simulink model "sample04_speed_pid"  (R2023a)
settings: Solver=ode1  StartTime=0.0  StopTime=inf  FixedStep=0.005  RelTol=1e-3  EnableMultiTasking=on
libraries: arduinolib x7, simulink x3, svdutilitieslib x1
settings Model: ExtModeTrigDuration=2  Creator=kawata  LastModifiedBy=kawata
settings SolverCC: AutoInsertRateTranBlk=on
settings DataIOCC: ReturnWorkspaceOutputs=off
settings OptimizationCC: EnhancedBackFolding=on  PassReuseOutputArgsAs=Individual arguments  ZeroExternalMemoryAtStartup=off  ZeroInternalMemoryAtStartup=off  MaxStackSize=64  OptimizeBlockOrder=speed  DifferentSizesBufferReuse=on  OptimizationCustomize=off  EfficientTunableParamExpr=on
settings DebuggingCC: ParameterTunabilityLossMsg=error
settings HardwareCC: ProdBitPerInt=16  ProdBitPerPointer=16  ProdBitPerSizeT=16  ProdBitPerPtrDiffT=16  ProdLargestAtomicFloat=None  ProdWordSize=8  ProdHWDeviceType=Atmel->AVR  UseEmbeddedCoderFeatures=off  UseSimulinkCoderFeatures=off
settings SFSimCC: MATLABDynamicMemAlloc=off
settings RTWCC: Description=Embedded Coder  SystemTargetFile=ert.tlc  HardwareBoard=Arduino Mega 2560  TemplateMakefile=ert_default_tmf  Toolchain=Arduino AVR  BuildConfiguration=Faster Runs  GPUComputeCapability=5.0
settings CodeAppCC: ForceParamTrailComments=on  IgnoreCustomStorageClasses=off  OperatorAnnotations=on  SimulinkDataObjDesc=on  SFDataObjDesc=on  InsertBlockDesc=on
settings ERTTargetCC: SupportContinuousTime=on  SupportNonInlinedSFcns=on  SupportVariableSizeSignals=on  ExtModeTransport=3  ExtModeStaticAlloc=on  ExtModeAutomaticAllocSize=off  ExtModeStaticAllocSize=2048  ExtModeMexFile=ext_xcp  ExtModeIntrfLevel=Level2 - Open

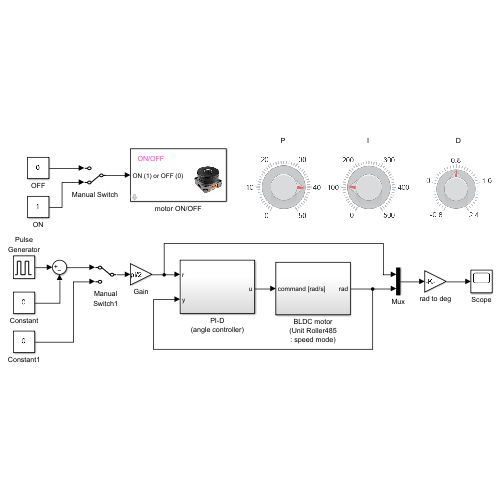
[thumbnail: Simulink's stored preview of the top-level diagram]
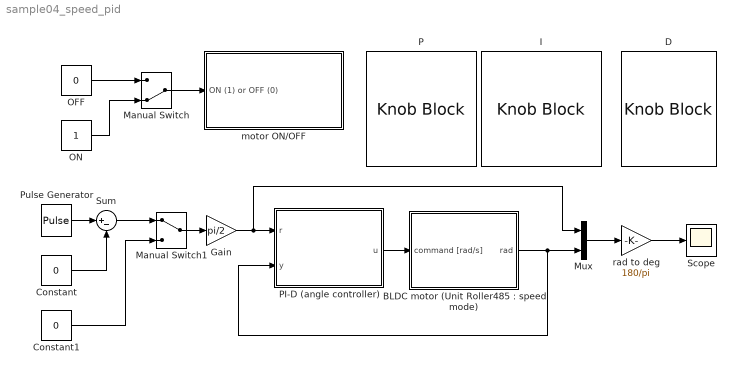
== system sample04_speed_pid ==
  "BLDC motor (Unit Roller485 : speed mode)" : Subsystem
  Constant : Constant  Value=0
  Constant1 : Constant  Value=0
  D : KnobBlock  LabelPosition=Hide  ScaleMin=-0.8  ScaleMax=2.4  TickInterval=0.8
  Gain : Gain  Gain=pi/2
  I : KnobBlock  LabelPosition=Hide  ScaleMax=500  TickInterval=100
  Manual Switch1 : ManualSwitch
  Manual Switch : ManualSwitch  CurrentSetting=0
  Mux : Mux  Inputs=2
  OFF : Constant  Value=0
  ON : Constant
  P : KnobBlock  LabelPosition=Hide  ScaleMax=50  TickInterval=10
  PI-D (angle controller) : Subsystem
  Pulse Generator : DiscretePulseGenerator  PulseType=Time based  Period=4  PulseWidth=50  PhaseDelay=1
  Scope : Scope
  Sum : Sum  Inputs=|+-
  motor ON/OFF : Subsystem  mask{I2CAddress=0x64}
      mask prompts: I2CAddress "I2C Address"
      mask help:
      | 0: motor off
      | 1: motor on
      mask DialogControl ParameterGroupVar Prompt: パラメーター
      mask Display:
      | image('roller485.png', [55,10,75,56]);
      | color('magenta');
      | text(10, 60, 'ON/OFF');
  rad to deg : Gain  Gain=180/pi
  wires:
  Manual Switch/1 -> motor ON/OFF/1(ON (1) or OFF (0))
  OFF/1 -> Manual Switch/1
  ON/1 -> Manual Switch/2
  Constant/1 -> Sum/2
  Pulse Generator/1 -> Sum/1
  Mux/1 -> rad to deg/1
  PI-D (angle controller)/1(u) -> "BLDC motor (Unit Roller485 : speed mode)"/1(command [rad/s])
  Gain/1 -> PI-D (angle controller)/1(r), Mux/1
  "BLDC motor (Unit Roller485 : speed mode)"/1(rad) -> PI-D (angle controller)/2(y), Mux/2
  rad to deg/1 -> Scope/1
  Manual Switch1/1 -> Gain/1
  Sum/1 -> Manual Switch1/1
  Constant1/1 -> Manual Switch1/2

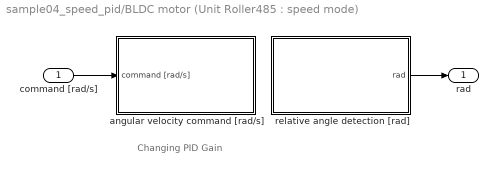
== system sample04_speed_pid/BLDC motor (Unit Roller485 : speed mode) ==
  note: Changing PID Gain
  command [rad/s] : Inport
  angular velocity command [rad/s] : Subsystem  mask(angular velocity command [rad/s]){I2CAddress=0x64, set_time=0, speed_P=2, speed_I=0, speed_D=600}
      mask prompts: I2CAddress "I2C Address"; set_time "Set Time"; speed_P "P"; speed_I "I"; speed_D "D"
      mask help:
      | speed mode
      | ---------------------------------
      | default value (PID gain of speed controller)
      |  P: 15
      |  I: 0.0001
      |  D: 400
      | ---------------------------------
      | If t ≤ set_time, then PID gain can be set.
      mask DialogControl ParameterGroupVar Prompt: パラメーター
      mask Display:
      | image('roller485.png', [55,10,75,56]);
      | color('green');
      | text(10, 60, 'speed control');
      | text(17, 22, '# mode setting');
      | text(17, 10, '# PID gain setting');
  relative angle detection [rad] : Subsystem  mask{I2CAddress=0x64, sample_time=0.005}
      mask prompts: I2CAddress "I2C Address"; sample_time "Sample Time"
      mask DialogControl ParameterGroupVar Prompt: パラメーター
      mask Display:
      | image('roller485.png', [30,10,75,56]);
      | color('blue');
      | text(10, 60, 'relative angle detection');
  rad : Outport
  wires:
  command [rad/s]/1 -> angular velocity command [rad/s]/1(command [rad/s])
  relative angle detection [rad]/1(rad) -> rad/1

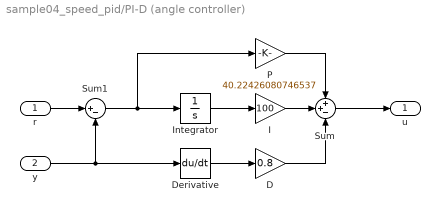
== system sample04_speed_pid/PI-D (angle controller) ==
  r : Inport
  y : Inport  Port=2
  D : Gain  Gain=0.8
  Derivative : Derivative
  I : Gain  Gain=100
  Integrator : Integrator
  P : Gain  Gain=40.22426080746537
  Sum : Sum  Inputs=++-
  Sum1 : Sum  Inputs=|+-
  u : Outport
  wires:
  Sum/1 -> u/1
  P/1 -> Sum/1
  I/1 -> Sum/2
  D/1 -> Sum/3
  Derivative/1 -> D/1
  Integrator/1 -> I/1
  r/1 -> Sum1/1
  Sum1/1 -> P/1, Integrator/1
  y/1 -> Sum1/2, Derivative/1

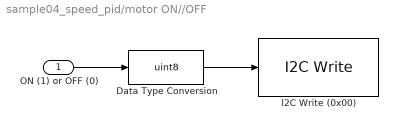
== system sample04_speed_pid/motor ON//OFF ==
  ON (1) or OFF (0) : Inport
  Data Type Conversion : DataTypeConversion  OutDataTypeStr=uint8  SaturateOnIntegerOverflow=off  RndMeth=Floor
  I2C Write (0x00) : arduinolib/I2C Write  I2CModule=0  Mode=Master  SlaveAddress=I2CAddress  SlaveByteOrder=BigEndian  Direction=Transmitter  RegisterAddressMode=on  RegisterAddress=0x00  SlaveDataType=uint8  DataLength=1  NoAck=off  RepeatedStart=off  OutputStatus=off  blockPlatform=ARDUINO
  wires:
  Data Type Conversion/1 -> I2C Write (0x00)/1
  ON (1) or OFF (0)/1 -> Data Type Conversion/1

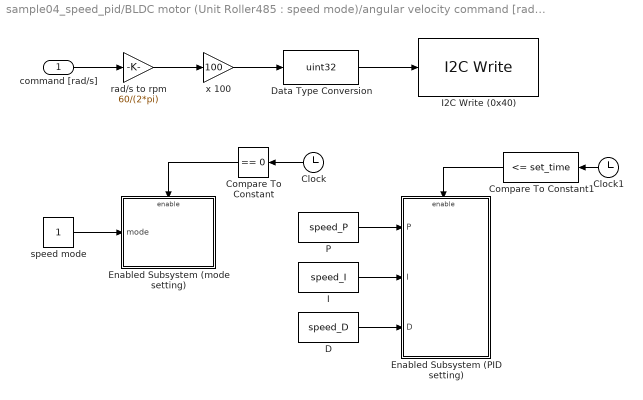
== system sample04_speed_pid/BLDC motor (Unit Roller485 : speed mode)/angular velocity command [rad//s] ==
  command [rad/s] : Inport
  "Clock " : Clock
  Clock1 : Clock
  Compare To Constant : simulink/Logic and Bit Operations/Compare To Constant  relop===  const=0  OutDataTypeStr=boolean
  Compare To Constant1 : simulink/Logic and Bit Operations/Compare To Constant  relop=<=  const=set_time  OutDataTypeStr=boolean
  D : Constant  Value=speed_D
  Data Type Conversion : DataTypeConversion  OutDataTypeStr=uint32  SaturateOnIntegerOverflow=off  RndMeth=Floor
  Enabled Subsystem (PID setting) : Subsystem  TreatAsAtomicUnit=on
  Enabled Subsystem (mode setting) : Subsystem  TreatAsAtomicUnit=on
  I : Constant  Value=speed_I
  I2C Write (0x40) : arduinolib/I2C Write  I2CModule=0  Mode=Master  SlaveAddress=I2CAddress  SlaveByteOrder=LittleEndian  Direction=Transmitter  RegisterAddressMode=on  RegisterAddress=0x40  SlaveDataType=uint8  DataLength=1  NoAck=off  RepeatedStart=off  OutputStatus=off  blockPlatform=ARDUINO
  P : Constant  Value=speed_P
  rad/s to rpm : Gain  Gain=60/(2*pi)
  speed mode : Constant
  x 100 : Gain  Gain=100
  wires:
  x 100/1 -> Data Type Conversion/1
  D/1 -> Enabled Subsystem (PID setting)/3(D)
  "Clock "/1 -> Compare To Constant/1
  Compare To Constant/1 -> Enabled Subsystem (mode setting)/Enable
  Compare To Constant1/1 -> Enabled Subsystem (PID setting)/Enable
  speed mode/1 -> Enabled Subsystem (mode setting)/1(mode)
  P/1 -> Enabled Subsystem (PID setting)/1(P)
  Clock1/1 -> Compare To Constant1/1
  I/1 -> Enabled Subsystem (PID setting)/2(I)
  Data Type Conversion/1 -> I2C Write (0x40)/1
  rad/s to rpm/1 -> x 100/1
  command [rad/s]/1 -> rad/s to rpm/1

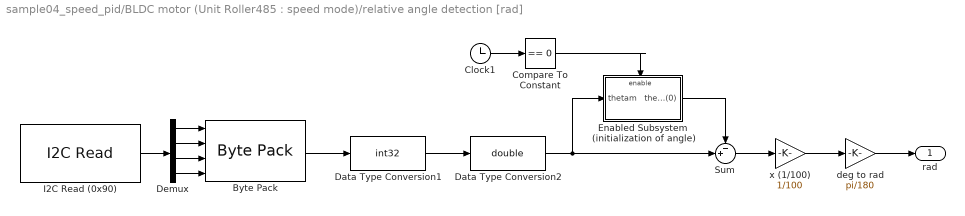
== system sample04_speed_pid/BLDC motor (Unit Roller485 : speed mode)/relative angle detection [rad] ==
  Byte Pack : svdutilitieslib/Byte Pack  maskPackedDataType=uint32  datatypes={'uint8','uint8','uint8','uint8'}  byteAlign=1  blockPlatform=arduinoert
  Clock1 : Clock
  Compare To Constant : simulink/Logic and Bit Operations/Compare To Constant  relop===  const=0  OutDataTypeStr=boolean
  Data Type Conversion1 : DataTypeConversion  OutDataTypeStr=int32  SaturateOnIntegerOverflow=off  RndMeth=Floor
  Data Type Conversion2 : DataTypeConversion  OutDataTypeStr=double  SaturateOnIntegerOverflow=off  RndMeth=Floor
  Demux : Demux
  Enabled Subsystem (initialization of angle) : Subsystem  TreatAsAtomicUnit=on
  I2C Read (0x90) : arduinolib/I2C Read  I2CModule=0  Mode=Master  SlaveAddress=0x64  SlaveByteOrder=BigEndian  Direction=Receiver  RegisterAddressMode=on  RegisterAddress=0x90  SlaveDataType=uint8  DataLength=4  NoAck=off  RepeatedStart=off  OutputStatus=off  blockPlatform=ARDUINO  SampleTime=sample_time
  Sum : Sum  Inputs=-+|
  deg to rad : Gain  Gain=pi/180
  x (1/100) : Gain  Gain=1/100
  rad : Outport
  wires:
  x (1/100)/1 -> deg to rad/1
  Clock1/1 -> Compare To Constant/1
  Compare To Constant/1 -> Enabled Subsystem (initialization of angle)/Enable
  Data Type Conversion2/1 -> Enabled Subsystem (initialization of angle)/1(thetam), Sum/2
  Enabled Subsystem (initialization of angle)/1(thetam(0)) -> Sum/1
  Sum/1 -> x (1/100)/1
  deg to rad/1 -> rad/1
  Demux/1 -> Byte Pack/1
  Demux/4 -> Byte Pack/4
  Demux/2 -> Byte Pack/2
  Byte Pack/1 -> Data Type Conversion1/1
  Data Type Conversion1/1 -> Data Type Conversion2/1
  Demux/3 -> Byte Pack/3
  I2C Read (0x90)/1 -> Demux/1

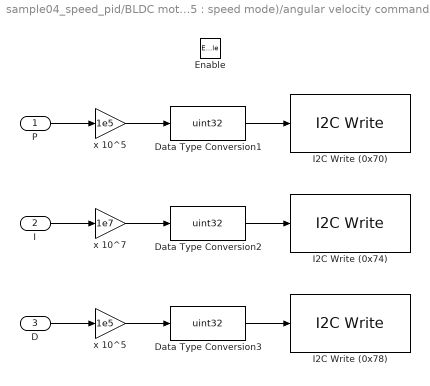
== system sample04_speed_pid/BLDC motor (Unit Roller485 : speed mode)/angular velocity command [rad//s]/Enabled Subsystem (PID setting) ==
  P : Inport
  I : Inport  Port=2
  D : Inport  Port=3
  Enable : EnablePort
  " x 10^5 " : Gain  Gain=1e5
  Data Type Conversion1 : DataTypeConversion  OutDataTypeStr=uint32  SaturateOnIntegerOverflow=off  RndMeth=Floor
  Data Type Conversion2 : DataTypeConversion  OutDataTypeStr=uint32  SaturateOnIntegerOverflow=off  RndMeth=Floor
  Data Type Conversion3 : DataTypeConversion  OutDataTypeStr=uint32  SaturateOnIntegerOverflow=off  RndMeth=Floor
  I2C Write (0x70) : arduinolib/I2C Write  I2CModule=0  Mode=Master  SlaveAddress=I2CAddress  SlaveByteOrder=LittleEndian  Direction=Transmitter  RegisterAddressMode=on  RegisterAddress=0x70  SlaveDataType=uint8  DataLength=1  NoAck=off  RepeatedStart=off  OutputStatus=off  blockPlatform=ARDUINO
  I2C Write (0x74) : arduinolib/I2C Write  I2CModule=0  Mode=Master  SlaveAddress=I2CAddress  SlaveByteOrder=LittleEndian  Direction=Transmitter  RegisterAddressMode=on  RegisterAddress=0x74  SlaveDataType=uint8  DataLength=1  NoAck=off  RepeatedStart=off  OutputStatus=off  blockPlatform=ARDUINO
  I2C Write (0x78) : arduinolib/I2C Write  I2CModule=0  Mode=Master  SlaveAddress=I2CAddress  SlaveByteOrder=LittleEndian  Direction=Transmitter  RegisterAddressMode=on  RegisterAddress=0x78  SlaveDataType=uint8  DataLength=1  NoAck=off  RepeatedStart=off  OutputStatus=off  blockPlatform=ARDUINO
  x 10^5 : Gain  Gain=1e5
  x 10^7 : Gain  Gain=1e7
  wires:
  " x 10^5 "/1 -> Data Type Conversion3/1
  x 10^7/1 -> Data Type Conversion2/1
  x 10^5/1 -> Data Type Conversion1/1
  Data Type Conversion1/1 -> I2C Write (0x70)/1
  Data Type Conversion3/1 -> I2C Write (0x78)/1
  Data Type Conversion2/1 -> I2C Write (0x74)/1
  D/1 -> " x 10^5 "/1
  I/1 -> x 10^7/1
  P/1 -> x 10^5/1

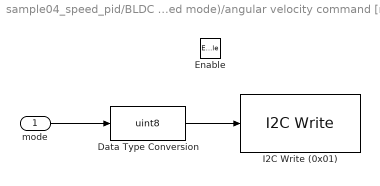
== system sample04_speed_pid/BLDC motor (Unit Roller485 : speed mode)/angular velocity command [rad//s]/Enabled Subsystem (mode setting) ==
  mode : Inport
  Enable : EnablePort
  Data Type Conversion : DataTypeConversion  OutDataTypeStr=uint8  SaturateOnIntegerOverflow=off  RndMeth=Floor
  I2C Write (0x01) : arduinolib/I2C Write  I2CModule=0  Mode=Master  SlaveAddress=I2CAddress  SlaveByteOrder=BigEndian  Direction=Transmitter  RegisterAddressMode=on  RegisterAddress=0x01  SlaveDataType=uint8  DataLength=1  NoAck=off  RepeatedStart=off  OutputStatus=off  blockPlatform=ARDUINO
  wires:
  mode/1 -> Data Type Conversion/1
  Data Type Conversion/1 -> I2C Write (0x01)/1

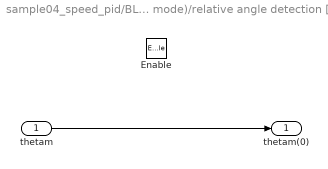
== system sample04_speed_pid/BLDC motor (Unit Roller485 : speed mode)/relative angle detection [rad]/Enabled Subsystem (initialization of angle) ==
  thetam : Inport
  Enable : EnablePort
  thetam(0) : Outport
  wires:
  thetam/1 -> thetam(0)/1
